simulink model "Exp_3_batch_12_simulation3"  (R2020a)
settings: Solver=VariableStepAuto  StartTime=0.0  StopTime=20  RelTol=1e-3
settings Model: Creator=sundaram bhupathi  LastModifiedBy=sundaram bhupathi

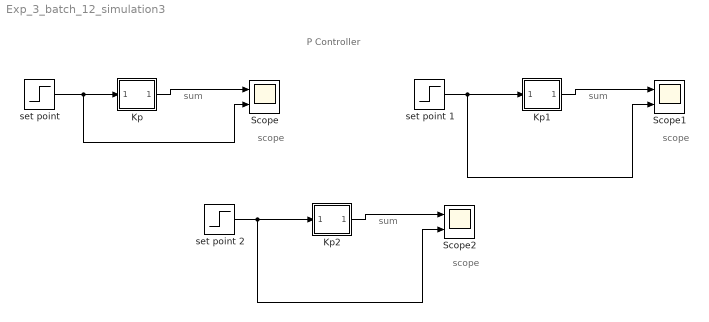
== system Exp_3_batch_12_simulation3 ==
  note: scope
  note: sum
  note: P Controller
  note: sum
  note: scope
  note: scope
  note: sum
  Kp : Subsystem
  Kp1 : Subsystem
  Kp2 : Subsystem
  Scope : Scope  NumInputPorts=2
  Scope1 : Scope  NumInputPorts=2
  Scope2 : Scope  NumInputPorts=2
  set point : Step  Before=1  SampleTime=0
  set point 1 : Step  Before=1  SampleTime=0
  set point 2 : Step  Before=1  SampleTime=0
  wires:
  Kp/1(Out1) -> Scope/1
  Kp2/1(Out1) -> Scope2/1
  set point 2/1 -> Scope2/2, Kp2/1(In1)
  Kp1/1(Out1) -> Scope1/1
  set point 1/1 -> Scope1/2, Kp1/1(In1)
  set point/1 -> Scope/2, Kp/1(In1)

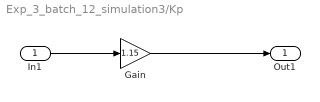
== system Exp_3_batch_12_simulation3/Kp ==
  In1 : Inport
  Gain : Gain  Gain=1.15
  Out1 : Outport
  wires:
  In1/1 -> Gain/1
  Gain/1 -> Out1/1

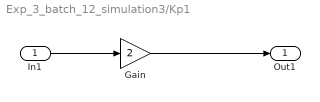
== system Exp_3_batch_12_simulation3/Kp1 ==
  In1 : Inport
  Gain : Gain  Gain=2
  Out1 : Outport
  wires:
  In1/1 -> Gain/1
  Gain/1 -> Out1/1

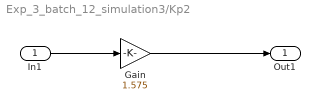
== system Exp_3_batch_12_simulation3/Kp2 ==
  In1 : Inport
  Gain : Gain  Gain=1.575
  Out1 : Outport
  wires:
  In1/1 -> Gain/1
  Gain/1 -> Out1/1
